simulink model "radia_electromagnet"  (R2026a)
settings: Solver=FixedStepDiscrete  StopTime=0.20000000000000001  FixedStep=0.10000000000000001
model workspace (MAT data in the model file):
  radia_electromagnet_adjoint_runner = radia.topopt.AdjointRunner
  radia_electromagnet_adjoint_runner.InitialDesign = [0.5; 0.5; 0.5; 0.5]
  radia_electromagnet_adjoint_runner.EvaluateFcn : function handle (value not decoded)
  radia_electromagnet_adjoint_runner.Options.StepTolerance = 0.0005
  radia_electromagnet_adjoint_runner.Options.OptimalityTolerance = 2e-05
  radia_electromagnet_adjoint_runner.Options.ConstraintTolerance = 1e-08
  radia_electromagnet_adjoint_runner.Options.LowerBounds = [0; 0; 0; 0]
  radia_electromagnet_adjoint_runner.Options.UpperBounds = [1; 1; 1; 1]
  radia_electromagnet_adjoint_runner.Options.MoveLimit = [0.2; 0.2; 0.2; 0.2]
  radia_electromagnet_adjoint_runner.Options.MaxIterations = 80
  radia_electromagnet_adjoint_runner.Metadata.domain = "electromagnet-topology"
  radia_electromagnet_adjoint_runner.Metadata.formulation = "vim-density-adjoint"
  radia_electromagnet_adjoint_runner.Metadata.state_equation = "A(rho)*m=b(rho)"
  radia_electromagnet_adjoint_runner.Metadata.gradient = "one-state-one-adjoint"
  radia_electromagnet_adjoint_runner.Metadata.design_count = 4
  radia_electromagnet_adjoint_runner.Metadata.response_count = 4
  radia_electromagnet_adjoint_runner.Metadata.volume_fraction_limit = 0.5
  radia_electromagnet_adjoint_runner.Metadata.element_volumes = [1; 1; 1; 1]
  radia_electromagnet_adjoint_runner.Metadata.penalization_power = 1
  radia_electromagnet_adjoint_runner.Metadata.python_per_step = 0
  radia_electromagnet_adjoint_runner.Metadata.reference_density = [0.9; 0.7; 0.3; 0.1]
  radia_electromagnet_adjoint_runner.Metadata.source = "preassembled-electromagnet-reference-operator"
settings Model: Creator=Administrator  LastModifiedBy=Administrator

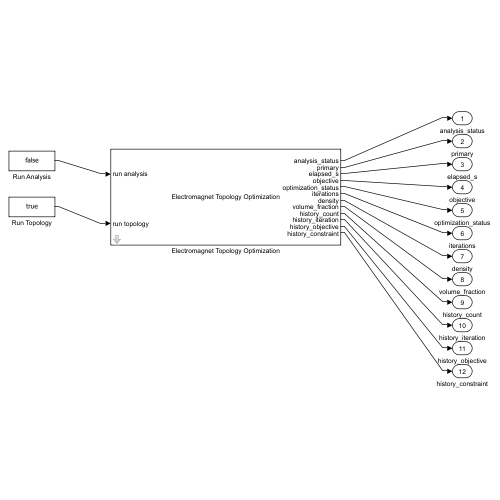
[thumbnail: Simulink's stored preview of the top-level diagram]
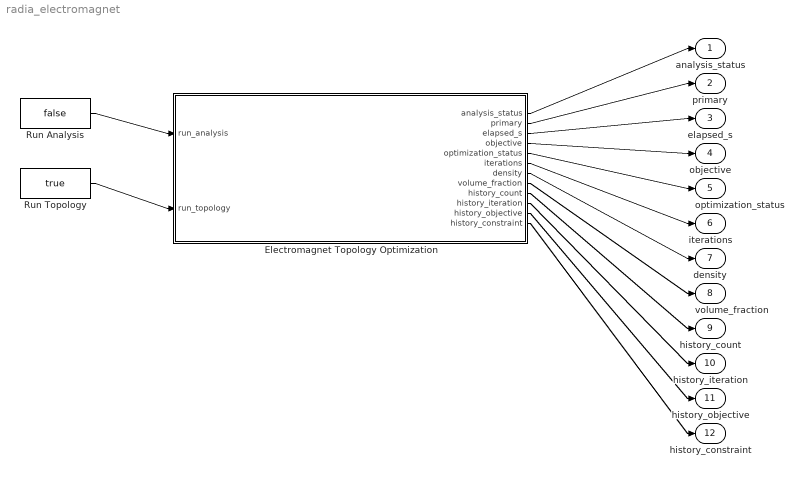
== system radia_electromagnet ==
  Electromagnet Topology Optimization : Subsystem  Tag=RadiaElectromagnetTopology  mask{config_file='', run_root='C:\temp\radia_simulink', timeout_s=3600, python_executable='python', radia_electromagnet_adjoint_runner=radia_electromagnet_adjoint_runner, solver=mma, sample_time_s=0.10000000000000001, history_capacity=96}
      mask prompts: config_file "Analysis configuration JSON"; run_root "Run artifact root"; timeout_s "Timeout (s)"; python_executable "Python executable"; radia_electromagnet_adjoint_runner "Electromagnet adjoint runner"; solver "Optimizer"; sample_time_s "Sample time (s)"; history_capacity "History capacity"
      mask help: Electromagnet batch analysis plus density topology optimization with one VIM state solve, one adjoint solve, and MMA/SQP.
      mask init:
      | radia.simulink.configureElectromagnetOptimizationSubsystem(gcb);
      mask TypeOptions solver: mma | sqp
      mask Display: disp('Electromagnet Topology Optimization');port_label('input',1,'run analysis');port_label('input',2,'run topology');port_label('output',1,'analysis_status');port_label('output',2,'primary');port_label('output',3,'elapsed_s');port_label('output',4,'objective');port_label('output',5,'optimization_status');port_label('output',6,'iterations');port_label('output',7,'density');port_label('output',8,'volume_fraction');port_label('output',9,'history_count');port_label('output',10,'history_iteration');port_label('output',11,'history_objective');port_label('output',12,'history_constraint');
  Run Analysis : Constant  Value=false  OutDataTypeStr=boolean
  Run Topology : Constant  Value=true  OutDataTypeStr=boolean
  analysis_status : Outport
  primary : Outport  Port=2
  elapsed_s : Outport  Port=3
  objective : Outport  Port=4
  optimization_status : Outport  Port=5
  iterations : Outport  Port=6
  density : Outport  Port=7
  volume_fraction : Outport  Port=8
  history_count : Outport  Port=9
  history_iteration : Outport  Port=10
  history_objective : Outport  Port=11
  history_constraint : Outport  Port=12
  wires:
  Run Analysis/1 -> Electromagnet Topology Optimization/1(run_analysis)
  Run Topology/1 -> Electromagnet Topology Optimization/2(run_topology)
  Electromagnet Topology Optimization/1(analysis_status) -> analysis_status/1
  Electromagnet Topology Optimization/2(primary) -> primary/1
  Electromagnet Topology Optimization/3(elapsed_s) -> elapsed_s/1
  Electromagnet Topology Optimization/4(objective) -> objective/1
  Electromagnet Topology Optimization/5(optimization_status) -> optimization_status/1
  Electromagnet Topology Optimization/6(iterations) -> iterations/1
  Electromagnet Topology Optimization/7(density) -> density/1
  Electromagnet Topology Optimization/8(volume_fraction) -> volume_fraction/1
  Electromagnet Topology Optimization/9(history_count) -> history_count/1
  Electromagnet Topology Optimization/10(history_iteration) -> history_iteration/1
  Electromagnet Topology Optimization/11(history_objective) -> history_objective/1
  Electromagnet Topology Optimization/12(history_constraint) -> history_constraint/1

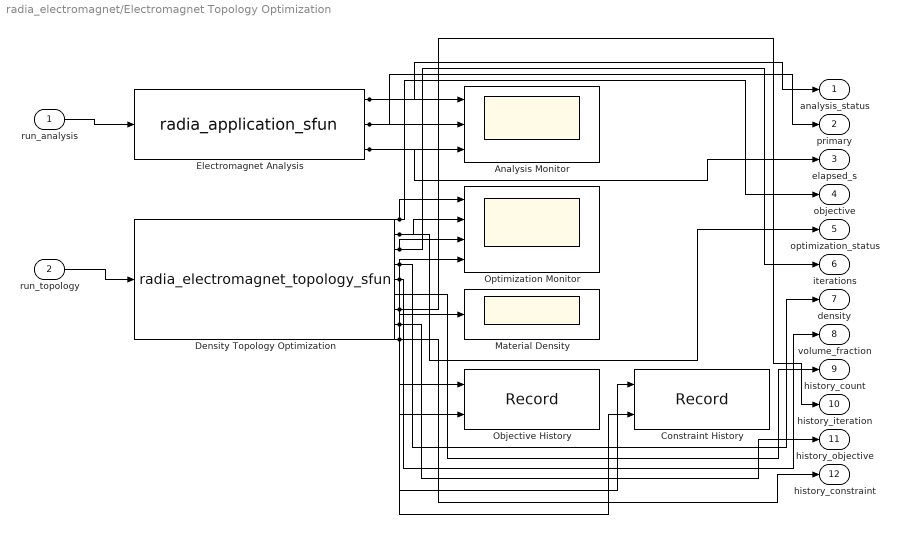
== system radia_electromagnet/Electromagnet Topology Optimization ==
  run_analysis : Inport  OutDataTypeStr=boolean
  run_topology : Inport  Port=2  OutDataTypeStr=boolean
  Analysis Monitor : Scope  NumInputPorts=3
  Constraint History : Record  NumPorts=2.0  FileSettingsInternal="{\"entries\":[{\"content\":{\"excelSettings\":{\"content\":{},\"type\":\"Streamout.ExcelSettings\"},\"parquetSettings\":{\"content\":{},\"type\":\"Streamout.ParquetSettings\"}},\"type\":\"Streamout.FileSettingStorage\",\"uuid\":\"\"}],\"packageUris\":[\"http:\\/\\/schema.mathworks.com\\/mf0\\/streamout_blocks\\/R2020a\"],\"version\":\"1.0\"}"  FrameSettings=[0, 0]  Layout=[1 1]  SignalsInternal="{\"entries\":[{\"content\":{\"signals\":[{\"content\":{\"blockPath\":[],\"dimensions\":[1],\"domain\":\"\",\"lineColor\":\"#a2142f\",\"plots\":[ 1 ],\"port\":1,\"signalID\":1,\"signalName\":\"XY Graph:1\"},\"type\":\"RecordBlkView.Signal\",\"uuid\":\"\"},{\"content\":{\"blockPath\":[],\"dimensions\":[1],\"domain\":\"\",\"lineColor\":\"#139fff\",\"plots\":[ 1 ],\"port\":2,\"signalID\":2,\"signalName\":\"XY Graph:2\"},\"type\":\"RecordBlkView.Signal\",\"uuid\":\"\"}]},\"type\":\"RecordBlkView.InputSignals\",\"uuid\":\"\"}],\"packageUris\":[\"http:\\/\\/schema.mathworks.com\\/mf0\\/streamout_blocks\\/R2020a\"],\"version\":\"1.0\"}"  VisualizationBindings="{\"xyplotplugin\":{\"info\":[{\"series\":[{\"bindingParametersList\":[{\"parameter\":\"X-Axis\",\"signalID\":1,\"signalName\":\"XY Graph:1\"},{\"parameter\":\"Y-Axis\",\"signalID\":2,\"signalName\":\"XY Graph:2\"}],\"seriesID\":0}],\"subplotID\":1}]}}"  CompatibilityTag=XY
  Density Topology Optimization : M-S-Function  FunctionName=radia_electromagnet_topology_sfun  Parameters=radia_electromagnet_adjoint_runner,0.10000000000000001,96
  Electromagnet Analysis : M-S-Function  FunctionName=radia_application_sfun  Parameters='em','','C:\temp\radia_simulink',3600,'python'
  Material Density : Scope
  Objective History : Record  NumPorts=2.0  FileSettingsInternal="{\"entries\":[{\"content\":{\"excelSettings\":{\"content\":{},\"type\":\"Streamout.ExcelSettings\"},\"parquetSettings\":{\"content\":{},\"type\":\"Streamout.ParquetSettings\"}},\"type\":\"Streamout.FileSettingStorage\",\"uuid\":\"\"}],\"packageUris\":[\"http:\\/\\/schema.mathworks.com\\/mf0\\/streamout_blocks\\/R2020a\"],\"version\":\"1.0\"}"  FrameSettings=[0, 0]  Layout=[1 1]  SignalsInternal="{\"entries\":[{\"content\":{\"signals\":[{\"content\":{\"blockPath\":[],\"dimensions\":[1],\"domain\":\"\",\"lineColor\":\"#a2142f\",\"plots\":[ 1 ],\"port\":1,\"signalID\":1,\"signalName\":\"XY Graph:1\"},\"type\":\"RecordBlkView.Signal\",\"uuid\":\"\"},{\"content\":{\"blockPath\":[],\"dimensions\":[1],\"domain\":\"\",\"lineColor\":\"#139fff\",\"plots\":[ 1 ],\"port\":2,\"signalID\":2,\"signalName\":\"XY Graph:2\"},\"type\":\"RecordBlkView.Signal\",\"uuid\":\"\"}]},\"type\":\"RecordBlkView.InputSignals\",\"uuid\":\"\"}],\"packageUris\":[\"http:\\/\\/schema.mathworks.com\\/mf0\\/streamout_blocks\\/R2020a\"],\"version\":\"1.0\"}"  VisualizationBindings="{\"xyplotplugin\":{\"info\":[{\"series\":[{\"bindingParametersList\":[{\"parameter\":\"X-Axis\",\"signalID\":1,\"signalName\":\"XY Graph:1\"},{\"parameter\":\"Y-Axis\",\"signalID\":2,\"signalName\":\"XY Graph:2\"}],\"seriesID\":0}],\"subplotID\":1}]}}"  CompatibilityTag=XY
  Optimization Monitor : Scope  NumInputPorts=4
  analysis_status : Outport
  primary : Outport  Port=2
  elapsed_s : Outport  Port=3
  objective : Outport  Port=4
  optimization_status : Outport  Port=5
  iterations : Outport  Port=6
  density : Outport  Port=7
  volume_fraction : Outport  Port=8
  history_count : Outport  Port=9
  history_iteration : Outport  Port=10
  history_objective : Outport  Port=11
  history_constraint : Outport  Port=12
  wires:
  run_analysis/1 -> Electromagnet Analysis/1
  run_topology/1 -> Density Topology Optimization/1
  Electromagnet Analysis/1 -> analysis_status/1, Analysis Monitor/1
  Electromagnet Analysis/2 -> primary/1, Analysis Monitor/2
  Electromagnet Analysis/3 -> elapsed_s/1, Analysis Monitor/3
  Density Topology Optimization/1 -> objective/1, Optimization Monitor/1
  Density Topology Optimization/2 -> optimization_status/1, Optimization Monitor/2
  Density Topology Optimization/3 -> iterations/1, Optimization Monitor/3
  Density Topology Optimization/4 -> density/1, Material Density/1
  Density Topology Optimization/5 -> volume_fraction/1, Optimization Monitor/4
  Density Topology Optimization/6 -> history_count/1
  Density Topology Optimization/7 -> history_iteration/1, Objective History/1, Constraint History/1
  Density Topology Optimization/8 -> history_objective/1, Objective History/2
  Density Topology Optimization/9 -> history_constraint/1, Constraint History/2
